simulink model "KrisztaSimulink"  (R2023b)
settings: Solver=VariableStepAuto  StartTime=0.0  StopTime=10^4  RelTol=1e-3
settings Model: Creator=kBen  LastModifiedBy=kBen
settings SolverCC: AlgebraicLoopSolver=TrustRegion

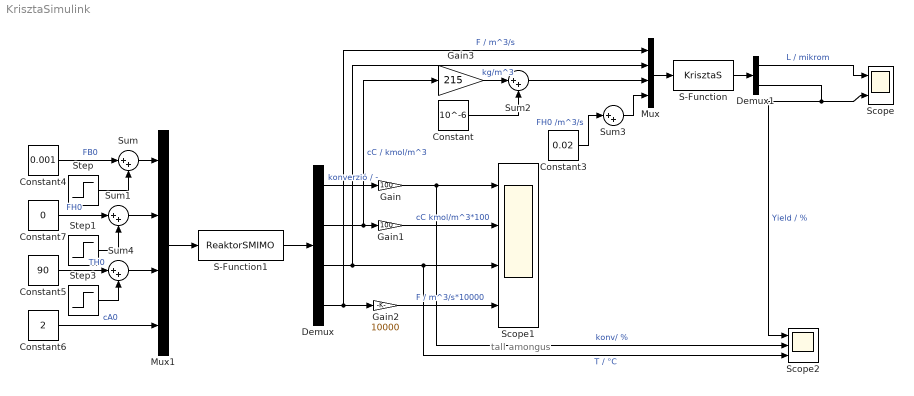
== system KrisztaSimulink ==
  note: tall amongus
  Constant : Constant  Value=10^-6
  Constant3 : Constant  Value=0.02
  Constant4 : Constant  Value=0.001
  Constant5 : Constant  Value=90
  Constant6 : Constant  Value=2
  Constant7 : Constant  Value=0
  Demux : Demux
  Demux1 : Demux  Outputs=2
  Gain : Gain  Gain=100
  Gain1 : Gain  Gain=100
  Gain2 : Gain  Gain=10000
  Gain3 : Gain  Gain=215
  Mux : Mux
  Mux1 : Mux
  S-Function : S-Function  FunctionName=KrisztaS  SFunctionDeploymentMode=off  EnableBusSupport=off
  S-Function1 : S-Function  FunctionName=ReaktorSMIMO  SFunctionDeploymentMode=off  EnableBusSupport=off
  Scope : Scope  NumInputPorts=2
  Scope1 : Scope  NumInputPorts=4
  Scope2 : Scope  NumInputPorts=3
  Step : Step  Time=5000  Before=0.0000  After=0.0000  SampleTime=0
  Step1 : Step  Time=0  After=0.01  SampleTime=0
  Step3 : Step  After=0  SampleTime=0
  Sum{,1..4} (5 alike) : Sum  Inputs=|++
  wires:
  Mux/1 -> S-Function/1
  S-Function/1 -> Demux1/1
  Constant3/1 -> Sum3/1  "FH0 /m^3/s"
  Mux1/1 -> S-Function1/1
  Constant4/1 -> Sum/1  "FB0"
  Constant7/1 -> Sum1/1  "FH0"
  S-Function1/1 -> Demux/1
  Demux/1 -> Gain/1  "konverzió / -"
  Demux/2 -> Gain3/1, Gain1/1  "cC / kmol/m^3"
  Demux/3 -> Mux/2, Scope2/3, Scope1/3  "T / °C"
  Demux/4 -> Mux/1, Gain2/1  "F / m^3/s"
  Demux1/1 -> Scope/1  "L / mikrom"
  Demux1/2 -> Scope2/1, Scope/2  "Yield / %"
  Gain/1 -> Scope2/2, Scope1/1  "konv/ %"
  Gain1/1 -> Scope1/2  "cC kmol/m^3*100"
  Gain2/1 -> Scope1/4  "F / m^3/s*10000"
  Sum/1 -> Mux1/1
  Step1/1 -> Sum1/2
  Sum1/1 -> Mux1/2
  Constant5/1 -> Sum4/1  "TH0"
  Constant6/1 -> Mux1/4  "cA0"
  Gain3/1 -> Sum2/1  "kg/m^3"
  Constant/1 -> Sum2/2
  Sum2/1 -> Mux/3
  Sum3/1 -> Mux/4
  Step/1 -> Sum/2
  Sum4/1 -> Mux1/3
  Step3/1 -> Sum4/2
